simulink model "MCP_phase2_linear_simulink"  (R2020a)
settings: Solver=VariableStepAuto  StartTime=0.0  StopTime=500  RelTol=1e-3
settings Model: Creator=rafiee  LastModifiedBy=Lenovo
settings DataIOCC: ReturnWorkspaceOutputs=off
settings DebuggingCC: ArithmeticOperatorsInVariantConditions=warning
settings SFSimCC: SimUseLocalCustomCode=off  CustomCodeUndefinedFunction=UseInterfaceOnly
settings RTWCC: RTWUseLocalCustomCode=off
settings CodeAppCC: StateflowObjectComments=on

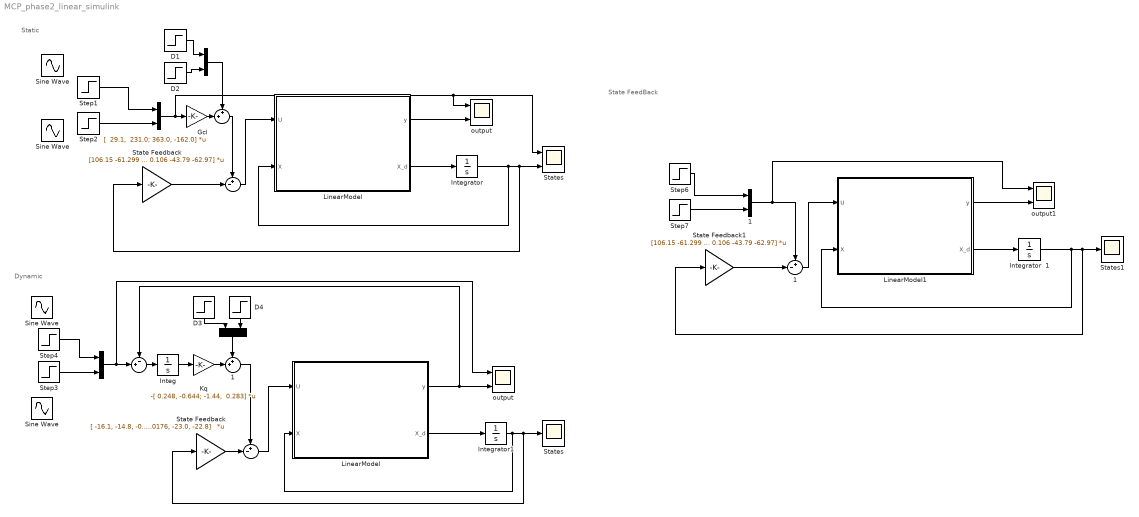
== system MCP_phase2_linear_simulink ==
  note: State FeedBack
  note: Dynamic
  note: Static
  " " : Sum  Inputs=+-|
  "   " : Concatenate
  "     " : Sum  Inputs=++|
  "       " : Concatenate
  "        " : Sum  Inputs=-+|
  "         " : Sum  Inputs=+-|
  "                                  " : Concatenate
  "                                                                   " : Concatenate
  "                  1" : Sum  Inputs=++|
  "   1" : Concatenate
  " 1" : Sum  Inputs=+-|
  D1 : Step  Time=250  After=4  SampleTime=0
  D2 : Step  Time=250  After=4  SampleTime=0
  D3 : Step  Time=250  After=5  SampleTime=0
  D4 : Step  Time=250  After=5  SampleTime=0
  Gcl : Gain  Gain="[  29.1,  231.0; 363.0, -162.0]"  Multiplication=Matrix(K*u)
  Integ : Integrator
  "Integrator  " : Integrator  InitialCondition=[0;0;0;0;0;0]
  Integrator  1 : Integrator  InitialCondition=[0;0;0;0;0;0]
  Integrator1 : Integrator  InitialCondition=[0;0;0;0;0;0]
  Kq : Gain  Gain="-[ 0.248, -0.644; -1.44,  0.283]"  Multiplication=Matrix(K*u)
  LinearModel : MATLAB Function  TreatAsAtomicUnit=on
  "LinearModel " : MATLAB Function  TreatAsAtomicUnit=on
  LinearModel1 : MATLAB Function  TreatAsAtomicUnit=on
  Sine Wave : Sin  SampleTime=0
  "Sine Wave " : Sin  SampleTime=0
  "Sine Wave  " : Sin  SampleTime=0
  "Sine Wave   " : Sin  SampleTime=0
  State Feedback : Gain  Gain=[106.15 -61.299 0.111 0.986 160.72 57.96; 169.55 189.92 1.35 0.106 -43.79 -62.97]  Multiplication=Matrix(K*u)
  "State Feedback " : Gain  Gain="[ -16.1, -14.8, -0.00412, -0.231,  27.5,  19.0;  55.9,  32.3,  -0.0575, 0.0176, -23.0, -22.8]"  Multiplication=Matrix(K*u)
  State Feedback1 : Gain  Gain=[106.15 -61.299 0.111 0.986 160.72 57.96; 169.55 189.92 1.35 0.106 -43.79 -62.97]  Multiplication=Matrix(K*u)
  States : Scope  NumInputPorts=2
  "States " : Scope
  States1 : Scope
  Step{1..4,6..7} (6 alike) : Step  SampleTime=0
  output : Scope  NumInputPorts=2
  "output " : Scope  NumInputPorts=2
  output1 : Scope  NumInputPorts=2
  wires:
  "   "/1 -> States/1, output/1, Gcl/1
  State Feedback/1 -> " "/2
  "Integrator  "/1 -> LinearModel/2(X), State Feedback/1, States/2
  LinearModel/1(y) -> output/2
  Integrator1/1 -> "LinearModel "/2(X), "State Feedback "/1, "States "/1
  "State Feedback "/1 -> "         "/2
  "LinearModel "/1(y) -> "        "/1, "output "/2
  "LinearModel "/2(X_d) -> Integrator1/1
  "         "/1 -> "LinearModel "/1(U)
  "       "/1 -> "output "/1, "        "/2
  "        "/1 -> Integ/1
  Integ/1 -> Kq/1
  Kq/1 -> "                  1"/2
  D3/1 -> "                                  "/1
  "                                  "/1 -> "                  1"/1
  "                  1"/1 -> "         "/1
  D1/1 -> "                                                                   "/1
  D2/1 -> "                                                                   "/2
  " "/1 -> LinearModel/1(U)
  "                                                                   "/1 -> "     "/1
  D4/1 -> "                                  "/2
  LinearModel/2(X_d) -> "Integrator  "/1
  Gcl/1 -> "     "/2
  "     "/1 -> " "/1
  LinearModel1/2(X_d) -> Integrator  1/1
  " 1"/1 -> LinearModel1/1(U)
  Integrator  1/1 -> LinearModel1/2(X), States1/1, State Feedback1/1
  LinearModel1/1(y) -> output1/2
  State Feedback1/1 -> " 1"/2
  Step7/1 -> "   1"/2
  Step6/1 -> "   1"/1
  "   1"/1 -> output1/1, " 1"/1
  Step1/1 -> "   "/1
  Step2/1 -> "   "/2
  Step4/1 -> "       "/1
  Step3/1 -> "       "/2

== matlab function MCP_phase2_linear_simulink/LinearModel  ==
  data: U input; y output; X input; X_d output
function [y,X_d]  = linear_plant(U,X)
A = [ -0.0189,  0.029,      0, 0.00306,       0,       0;
       0, -0.029, 0.0065,       0,       0,       0;
       0,      0, -0.476,       0,       0,       0;
       0,      0,      0,    -0.5,       0,       0;
       0,      0, 0.0035,       0, -0.0191,  0.0349;
       0,      0,      0, 0.00714,       0, -0.0349];

B =[0,     0;
   0,     0;
   0, 0.476;
   0.5,     0;
   0,     0;
   0,     0];

C = [1.0, 0, 0, 0, 0, 0;
     0, 0, 0, 0, 1.0, 0];
X_d = A * X + B * U; 
y = C*X;

== matlab function MCP_phase2_linear_simulink/LinearModel ==
  data: U input; y output; X input; X_d output
function [y,X_d]  = linear_plant(U,X)
A = [ -0.0189,  0.029,      0, 0.00306,       0,       0;
       0, -0.029, 0.0065,       0,       0,       0;
       0,      0, -0.476,       0,       0,       0;
       0,      0,      0,    -0.5,       0,       0;
       0,      0, 0.0035,       0, -0.0191,  0.0349;
       0,      0,      0, 0.00714,       0, -0.0349];

B =[0,     0;
   0,     0;
   0, 0.476;
   0.5,     0;
   0,     0;
   0,     0];

C = [1.0, 0, 0, 0, 0, 0;
     0, 0, 0, 0, 1.0, 0];
X_d = A * X + B * U; 
y = C*X;

== matlab function MCP_phase2_linear_simulink/LinearModel1 ==
  data: U input; y output; X input; X_d output
function [y,X_d]  = linear_plant(U,X)
A = [ -0.0189,  0.029,      0, 0.00306,       0,       0;
       0, -0.029, 0.0065,       0,       0,       0;
       0,      0, -0.476,       0,       0,       0;
       0,      0,      0,    -0.5,       0,       0;
       0,      0, 0.0035,       0, -0.0191,  0.0349;
       0,      0,      0, 0.00714,       0, -0.0349];

B =[0,     0;
   0,     0;
   0, 0.476;
   0.5,     0;
   0,     0;
   0,     0];

C = [1.0, 0, 0, 0, 0, 0;
     0, 0, 0, 0, 1.0, 0];
X_d = A * X + B * U; 
y = C*X;
